simulink model "runCampusSim"  (Simulink 8.1)
settings: Solver=FixedStepDiscrete  StartTime=0.0  StopTime=Inf  FixedStep=900  RelTol=1e-3
libraries: CampusEnergyModeling x5, simulink x3
settings Model: Creator=wbernal  LastModifiedBy=wbernal
settings DebuggingCC: FcnCallInpInsideContextMsg=EnableAllAsWarning

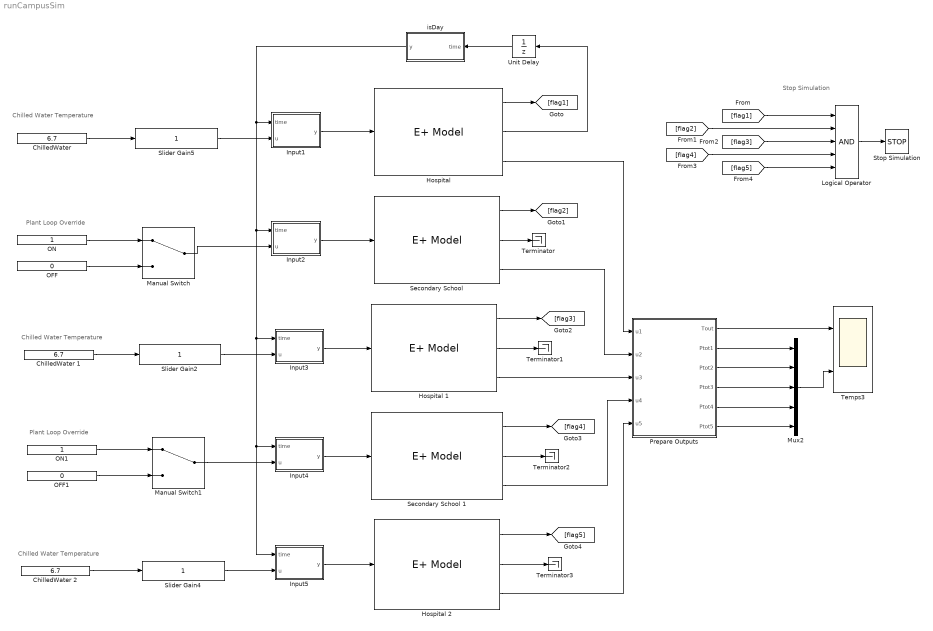
== system runCampusSim ==
  note: Stop Simulation
  note: Plant Loop Override
  note: Chilled Water Temperature
  note: Chilled Water Temperature
  note: Plant Loop Override
  note: Chilled Water Temperature
  ChilledWater : Constant  Value=6.7
  ChilledWater 1 : Constant  Value=6.7
  ChilledWater 2 : Constant  Value=6.7
  Hospital : CampusEnergyModeling/Buildings/E+ Model  progname='C:\EnergyPlusV8-0-0\RunEPlus.bat'  modelfile=[pwd '\Hospital\RefBldgHospitalNew2004_Chicago']  weatherfile='USA_IL_Chicago-OHare.Intl.AP.725300_TMY3'  workdir=[pwd '\Hospital\']  timeout=20e3  port=0  host=''  bcvtbdir=''  deltaT=900  noutputd=10
  Hospital 1 : CampusEnergyModeling/Buildings/E+ Model  progname='C:\EnergyPlusV8-0-0\RunEPlus.bat'  modelfile=[pwd '\Hospital1\RefBldgHospitalNew2004_Chicago']  weatherfile='USA_IL_Chicago-OHare.Intl.AP.725300_TMY3'  workdir=[pwd '\Hospital1\']  timeout=20e3  port=0  host=''  bcvtbdir=''  deltaT=900  noutputd=10
  Hospital 2 : CampusEnergyModeling/Buildings/E+ Model  progname='C:\EnergyPlusV8-0-0\RunEPlus.bat'  modelfile=[pwd '\Hospital2\RefBldgHospitalNew2004_Chicago']  weatherfile='USA_IL_Chicago-OHare.Intl.AP.725300_TMY3'  workdir=[pwd '\Hospital2\']  timeout=20e3  port=0  host=''  bcvtbdir=''  deltaT=900  noutputd=10
  Input1 : MATLAB Function  TreatAsAtomicUnit=on
  Input2 : MATLAB Function  TreatAsAtomicUnit=on
  Input3 : MATLAB Function  TreatAsAtomicUnit=on
  Input4 : MATLAB Function  TreatAsAtomicUnit=on
  Input5 : MATLAB Function  TreatAsAtomicUnit=on
  Logical Operator : Logic  Inputs=5  IconShape=distinctive  AllPortsSameDT=off  OutDataTypeStr=boolean
  Manual Switch : ManualSwitch
  Manual Switch1 : ManualSwitch
  Mux2 : Mux  Inputs=5
  OFF : Constant  Value=0
  OFF1 : Constant  Value=0
  ON : Constant
  ON1 : Constant
  Prepare Outputs : MATLAB Function  TreatAsAtomicUnit=on
  Secondary School : CampusEnergyModeling/Buildings/E+ Model  progname='C:\EnergyPlusV8-0-0\RunEPlus.bat'  modelfile=[pwd '\SecondarySchool\RefBldgSecondarySchoolNew2004_Chicago']  weatherfile='USA_IL_Chicago-OHare.Intl.AP.725300_TMY3'  workdir=[pwd '\SecondarySchool\']  timeout=20e3  port=0  host=''  bcvtbdir=''  deltaT=900  noutputd=19
  Secondary School 1 : CampusEnergyModeling/Buildings/E+ Model  progname='C:\EnergyPlusV8-0-0\RunEPlus.bat'  modelfile=[pwd '\SecondarySchool1\RefBldgSecondarySchoolNew2004_Chicago']  weatherfile='USA_IL_Chicago-OHare.Intl.AP.725300_TMY3'  workdir=[pwd '\SecondarySchool1\']  timeout=20e3  port=0  host=''  bcvtbdir=''  deltaT=900  noutputd=19
  Slider Gain2 : simulink/Math Operations/Slider Gain  low=0.75  gain=1  high=2
  Slider Gain4 : simulink/Math Operations/Slider Gain  low=0.75  gain=1  high=2
  Slider Gain5 : simulink/Math Operations/Slider Gain  low=0.75  gain=1  high=2
  Stop Simulation : Stop
  Temps3 : Scope  NumInputPorts=2
      settings: TimeRange=3000000  YMin=5~0  YMax=32.5~525000
  Terminator{,1..3} (4 alike) : Terminator
  Unit Delay : UnitDelay  SampleTime=-1
  isDay : Subsystem
  wires:
  Hospital/2 -> Unit Delay/1
  Input1/1(y) -> Hospital/1
  Input2/1(y) -> Secondary School/1
  isDay/1(y) -> Input1/1(time), Input2/1(time), Input3/1(time), Input4/1(time), Input5/1(time)
  Secondary School/2 -> Terminator/1
  Hospital/3 -> Prepare Outputs/1(u1)
  Logical Operator/1 -> Stop Simulation/1
  Hospital/1 -> [flag1]
  Secondary School/1 -> [flag2]
  [flag1] -> Logical Operator/1
  [flag2] -> Logical Operator/2
  Secondary School/3 -> Prepare Outputs/2(u2)
  Mux2/1 -> Temps3/2
  Prepare Outputs/1(Tout) -> Temps3/1
  Hospital 1/1 -> [flag3]
  Secondary School 1/1 -> [flag4]
  Hospital 2/1 -> [flag5]
  Hospital 1/2 -> Terminator1/1
  Secondary School 1/2 -> Terminator2/1
  Hospital 2/2 -> Terminator3/1
  Hospital 1/3 -> Prepare Outputs/3(u3)
  Secondary School 1/3 -> Prepare Outputs/4(u4)
  Hospital 2/3 -> Prepare Outputs/5(u5)
  [flag3] -> Logical Operator/3
  [flag4] -> Logical Operator/4
  [flag5] -> Logical Operator/5
  Prepare Outputs/2(Ptot1) -> Mux2/1
  Prepare Outputs/3(Ptot2) -> Mux2/2
  Prepare Outputs/4(Ptot3) -> Mux2/3
  Prepare Outputs/5(Ptot4) -> Mux2/4
  Prepare Outputs/6(Ptot5) -> Mux2/5
  Input4/1(y) -> Secondary School 1/1
  Input3/1(y) -> Hospital 1/1
  Input5/1(y) -> Hospital 2/1
  Manual Switch/1 -> Input2/2(u)
  ChilledWater 1/1 -> Slider Gain2/1
  Slider Gain2/1 -> Input3/2(u)
  ChilledWater 2/1 -> Slider Gain4/1
  Slider Gain4/1 -> Input5/2(u)
  ChilledWater/1 -> Slider Gain5/1
  Slider Gain5/1 -> Input1/2(u)
  ON/1 -> Manual Switch/1
  OFF/1 -> Manual Switch/2
  ON1/1 -> Manual Switch1/1
  OFF1/1 -> Manual Switch1/2
  Manual Switch1/1 -> Input4/2(u)
  Unit Delay/1 -> isDay/1(time)

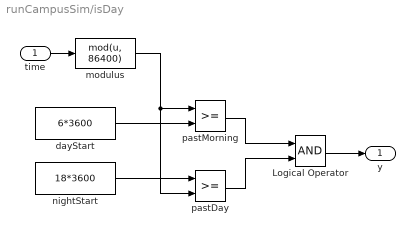
== system runCampusSim/isDay ==
  time : Inport
  Logical Operator : Logic  AllPortsSameDT=off  OutDataTypeStr=boolean
  dayStart : Constant  Value=6*3600
  modulus : MATLABFcn  MATLABFcn=mod(u, 86400)
  nightStart : Constant  Value=18*3600
  pastDay : RelationalOperator  OutDataTypeStr=boolean
  pastMorning : RelationalOperator  OutDataTypeStr=boolean
  y : Outport
  wires:
  time/1 -> modulus/1
  modulus/1 -> pastMorning/1, pastDay/2
  dayStart/1 -> pastMorning/2
  nightStart/1 -> pastDay/1
  pastMorning/1 -> Logical Operator/1
  pastDay/1 -> Logical Operator/2
  Logical Operator/1 -> y/1

== matlab function Input2 ==
  data: time input double; u input double; y output double
function y = fcn(time, u)

%% BEGIN - CONTROL
K1 = 0.001;
K2 = 0.0001;

% dayTime = mod(time, 86400);
% if (dayTime >= 6*3600) && (dayTime <= 18*3600)
%     if outputs1(2) + outputs2(2) > 9000
%         change = K1*(outputs1(2) + outputs2(2)-9000);
%         chilledWaterTempSch2 = chilledWaterTempSch2 + change;
%     else
%         change = K2*(outputs1(2) + outputs2(2)-9000);
%         chilledWaterTempSch2 = chilledWaterTempSch2 + change;
%     end
%     if chilledWaterTempSch2 < 7
%         chilledWaterTempSch2 = 7;
%     elseif chilledWaterTempSch2 > 10
%         chilledWaterTempSch2 = 10;
%     end
% end
% 
% 
% 
% inputs1 = [airTempSch roomTempSch chilledWaterTempSch1];
 
y = u(1);

== matlab function Input1 ==
  data: time input double; u input double; y output double
function y = fcn(time, u)


%% BEGIN - CONTROL
K1 = 0.001;
K2 = 0.0001;

% dayTime = mod(time, 86400);
% if (dayTime >= 6*3600) && (dayTime <= 18*3600)
%     if outputs1(2) + outputs2(2) > 9000
%         change = K1*(outputs1(2) + outputs2(2)-9000);
%         chilledWaterTempSch2 = chilledWaterTempSch2 + change;
%     else
%         change = K2*(outputs1(2) + outputs2(2)-9000);
%         chilledWaterTempSch2 = chilledWaterTempSch2 + change;
%     end
%     if chilledWaterTempSch2 < 7
%         chilledWaterTempSch2 = 7;
%     elseif chilledWaterTempSch2 > 10
%         chilledWaterTempSch2 = 10;
%     end
% end
% 
% 
% 
% inputs1 = [airTempSch roomTempSch chilledWaterTempSch1];
 
y = u;

== matlab function Prepare Outputs ==
  data: Tout output double; u1 input double; Ptot1 output double; u2 input double; Ptot2 output double; u3 input double; u4 input double; u5 input double; Ptot3 output double; Ptot4 output double; Ptot5 output double
function [Tout, Ptot1, Ptot2, Ptot3, Ptot4, Ptot5]  = PrepOutputs(u1, u2, u3, u4, u5)

Tout = u1(1);
Ptot1 = sum(u1(2:end));
Ptot2 = sum(u2(2:end));
Ptot3 = sum(u3(2:end));
Ptot4 = sum(u4(2:end));
Ptot5 = sum(u5(2:end));

== matlab function Input4 ==
  data: time input double; u input double; y output double
function y = fcn(time, u)


%% BEGIN - CONTROL
K1 = 0.001;
K2 = 0.0001;

% dayTime = mod(time, 86400);
% if (dayTime >= 6*3600) && (dayTime <= 18*3600)
%     if outputs1(2) + outputs2(2) > 9000
%         change = K1*(outputs1(2) + outputs2(2)-9000);
%         chilledWaterTempSch2 = chilledWaterTempSch2 + change;
%     else
%         change = K2*(outputs1(2) + outputs2(2)-9000);
%         chilledWaterTempSch2 = chilledWaterTempSch2 + change;
%     end
%     if chilledWaterTempSch2 < 7
%         chilledWaterTempSch2 = 7;
%     elseif chilledWaterTempSch2 > 10
%         chilledWaterTempSch2 = 10;
%     end
% end
% 
% 
% 
% inputs1 = [airTempSch roomTempSch chilledWaterTempSch1];
 
y = u;

== matlab function Input3 ==
  data: time input double; u input double; y output double
function y = fcn(time, u)


%% BEGIN - CONTROL
K1 = 0.001;
K2 = 0.0001;

% dayTime = mod(time, 86400);
% if (dayTime >= 6*3600) && (dayTime <= 18*3600)
%     if outputs1(2) + outputs2(2) > 9000
%         change = K1*(outputs1(2) + outputs2(2)-9000);
%         chilledWaterTempSch2 = chilledWaterTempSch2 + change;
%     else
%         change = K2*(outputs1(2) + outputs2(2)-9000);
%         chilledWaterTempSch2 = chilledWaterTempSch2 + change;
%     end
%     if chilledWaterTempSch2 < 7
%         chilledWaterTempSch2 = 7;
%     elseif chilledWaterTempSch2 > 10
%         chilledWaterTempSch2 = 10;
%     end
% end
% 
% 
% 
% inputs1 = [airTempSch roomTempSch chilledWaterTempSch1];
 
y = u;

== matlab function Input5 ==
  data: time input double; u input double; y output double
function y = fcn(time, u)


%% BEGIN - CONTROL
K1 = 0.001;
K2 = 0.0001;

% dayTime = mod(time, 86400);
% if (dayTime >= 6*3600) && (dayTime <= 18*3600)
%     if outputs1(2) + outputs2(2) > 9000
%         change = K1*(outputs1(2) + outputs2(2)-9000);
%         chilledWaterTempSch2 = chilledWaterTempSch2 + change;
%     else
%         change = K2*(outputs1(2) + outputs2(2)-9000);
%         chilledWaterTempSch2 = chilledWaterTempSch2 + change;
%     end
%     if chilledWaterTempSch2 < 7
%         chilledWaterTempSch2 = 7;
%     elseif chilledWaterTempSch2 > 10
%         chilledWaterTempSch2 = 10;
%     end
% end
% 
% 
% 
% inputs1 = [airTempSch roomTempSch chilledWaterTempSch1];
 
y = u;
